simulink model "Trí"  (R2019a)
settings: Solver=FixedStepAuto  StartTime=0.0  StopTime=15  FixedStep=0.01  RelTol=1e-3
model workspace (MATLAB code in the model file):
  | Assem_DataFile.m
undefined symbols (not defined in the file): smiData, X, Y, Z
libraries: sm_lib x272, simulink x8, nesl_utility x8
(part 6 of 6)

== system Trí/Sub_SW/SolidWorks/yoke_haft_arm_8_RIGID ==
  ReferenceFrame : sm_lib/Frames and Transforms/Reference Frame
  Solid : sm_lib/Body Elements/Solid  InertiaType=Custom  Mass=smiData.Solid(6).mass  MassUnits=kg  CenterOfMass=smiData.Solid(6).CoM  CenterOfMassUnits=mm  MomentsOfInertia=smiData.Solid(6).MoI  MomentsOfInertiaUnits=kg*mm^2  ProductsOfInertia=smiData.Solid(6).PoI  ProductsOfInertiaUnits=kg*mm^2  BasedOnType=Density  Density=1000  DensityUnits=kg/m^3  DoExposeReferenceFrame=on  SerializedFrames=<Frames/>  GraphicType=FromGeometry  MarkerShape=Sphere  MarkerSize=10  GraphicVisPropType=SimpleVisualProperties  GraphicDiffuseColor=smiData.Solid(6).color  GraphicSpecularColor=[0.5 0.5 0.5 1.0]  GraphicAmbientColor=[0.15 0.15 0.15 1.0]  GraphicEmissiveColor=[0.0 0.0 0.0 1.0]  GraphicShininess=75  GraphicOpacity=smiData.Solid(6).opacity  GeometryShape=FromFile  RectangleSize=[1 1]  RectangleSizeUnits=m  BrickDimensions=[1 1 1]  BrickDimensionUnits=m  CylinderRadius=1  CylinderRadiusUnits=m  CylinderLength=1  CylinderLengthUnits=m  SphereRadius=1  SphereRadiusUnits=m  EllipsoidRadii=[1 1 1]  EllipsoidRadiiUnits=m  ExtrusionCrossSection=[1 1; -1 1; -1 -1; 1 -1]  ExtrusionCrossSectionUnits=m  ExtrusionLength=1  ExtrusionLengthUnits=m  PolygonNumSides=3  PolygonOuterRadius=1  PolygonOuterRadiusUnits=m  ExtGeomFileType=STEP  ExtGeomFileName=yoke haft arm_Default_sldprt.STEP  ExtGeomFileUnits=m  RevolutionCrossSection=[1 1; 1 -1; 2 -1; 2 1]  RevolutionCrossSectionUnits=m  RevolutionExtent=Full  RevolutionAngle=180  RevolutionAngleUnits=deg
  Transform : sm_lib/Frames and Transforms/Rigid Transform  TranslationMethod=Cartesian  TranslationStandardOffset=0  TranslationLengthUnit=mm  TranslationStandardAxis=+Z  TranslationCartesianOffset=smiData.RigidTransform(66).translation  TranslationROffset=0  TranslationROffsetUnits=m  TranslationZOffset=0  TranslationZOffsetUnits=m  TranslationThetaOffset=0  TranslationThetaOffsetUnits=deg  RotationMethod=ArbitraryAxis  RotationAngleUnits=rad  RotationStandardAxis=+Z  RotationAngle=smiData.RigidTransform(66).angle  RotationArbitraryAxis=smiData.RigidTransform(66).axis  FollAlignAxisA=+X  BaseAlignAxisA=+Y  FollAlignAxisB=+Y  BaseAlignAxisB=+Z  RotationSequenceAxes=FollowerAxes  RotationSequence=XYX  RotationSequenceAngles=[0 0 0]  RotationSequenceAnglesUnits=deg  RotationMatrix=[1 0 0; 0 1 0; 0 0 1]
  Transform1 : sm_lib/Frames and Transforms/Rigid Transform  TranslationMethod=Cartesian  TranslationStandardOffset=0  TranslationLengthUnit=mm  TranslationStandardAxis=+Z  TranslationCartesianOffset=smiData.RigidTransform(121).translation  TranslationROffset=0  TranslationROffsetUnits=m  TranslationZOffset=0  TranslationZOffsetUnits=m  TranslationThetaOffset=0  TranslationThetaOffsetUnits=deg  RotationMethod=ArbitraryAxis  RotationAngleUnits=rad  RotationStandardAxis=+Z  RotationAngle=smiData.RigidTransform(121).angle  RotationArbitraryAxis=smiData.RigidTransform(121).axis  FollAlignAxisA=+X  BaseAlignAxisA=+Y  FollAlignAxisB=+Y  BaseAlignAxisB=+Z  RotationSequenceAxes=FollowerAxes  RotationSequence=XYX  RotationSequenceAngles=[0 0 0]  RotationSequenceAnglesUnits=deg  RotationMatrix=[1 0 0; 0 1 0; 0 0 1]
  F1 : PMIOPort  Side=Left
  F : PMIOPort  Port=2  Side=Left
  connections:
  Solid/RConn1 -- ReferenceFrame/RConn1 -- Transform/LConn1 -- Transform1/LConn1
  Transform/RConn1 -- F/RConn1
  Transform1/RConn1 -- F1/RConn1

== system Trí/Sub_SW/SolidWorks/yoke_haft_arm_9_RIGID ==
  ReferenceFrame : sm_lib/Frames and Transforms/Reference Frame
  Solid : sm_lib/Body Elements/Solid  InertiaType=Custom  Mass=smiData.Solid(6).mass  MassUnits=kg  CenterOfMass=smiData.Solid(6).CoM  CenterOfMassUnits=mm  MomentsOfInertia=smiData.Solid(6).MoI  MomentsOfInertiaUnits=kg*mm^2  ProductsOfInertia=smiData.Solid(6).PoI  ProductsOfInertiaUnits=kg*mm^2  BasedOnType=Density  Density=1000  DensityUnits=kg/m^3  DoExposeReferenceFrame=on  SerializedFrames=<Frames/>  GraphicType=FromGeometry  MarkerShape=Sphere  MarkerSize=10  GraphicVisPropType=SimpleVisualProperties  GraphicDiffuseColor=smiData.Solid(6).color  GraphicSpecularColor=[0.5 0.5 0.5 1.0]  GraphicAmbientColor=[0.15 0.15 0.15 1.0]  GraphicEmissiveColor=[0.0 0.0 0.0 1.0]  GraphicShininess=75  GraphicOpacity=smiData.Solid(6).opacity  GeometryShape=FromFile  RectangleSize=[1 1]  RectangleSizeUnits=m  BrickDimensions=[1 1 1]  BrickDimensionUnits=m  CylinderRadius=1  CylinderRadiusUnits=m  CylinderLength=1  CylinderLengthUnits=m  SphereRadius=1  SphereRadiusUnits=m  EllipsoidRadii=[1 1 1]  EllipsoidRadiiUnits=m  ExtrusionCrossSection=[1 1; -1 1; -1 -1; 1 -1]  ExtrusionCrossSectionUnits=m  ExtrusionLength=1  ExtrusionLengthUnits=m  PolygonNumSides=3  PolygonOuterRadius=1  PolygonOuterRadiusUnits=m  ExtGeomFileType=STEP  ExtGeomFileName=yoke haft arm_Default_sldprt.STEP  ExtGeomFileUnits=m  RevolutionCrossSection=[1 1; 1 -1; 2 -1; 2 1]  RevolutionCrossSectionUnits=m  RevolutionExtent=Full  RevolutionAngle=180  RevolutionAngleUnits=deg
  Transform : sm_lib/Frames and Transforms/Rigid Transform  TranslationMethod=Cartesian  TranslationStandardOffset=0  TranslationLengthUnit=mm  TranslationStandardAxis=+Z  TranslationCartesianOffset=smiData.RigidTransform(55).translation  TranslationROffset=0  TranslationROffsetUnits=m  TranslationZOffset=0  TranslationZOffsetUnits=m  TranslationThetaOffset=0  TranslationThetaOffsetUnits=deg  RotationMethod=ArbitraryAxis  RotationAngleUnits=rad  RotationStandardAxis=+Z  RotationAngle=smiData.RigidTransform(55).angle  RotationArbitraryAxis=smiData.RigidTransform(55).axis  FollAlignAxisA=+X  BaseAlignAxisA=+Y  FollAlignAxisB=+Y  BaseAlignAxisB=+Z  RotationSequenceAxes=FollowerAxes  RotationSequence=XYX  RotationSequenceAngles=[0 0 0]  RotationSequenceAnglesUnits=deg  RotationMatrix=[1 0 0; 0 1 0; 0 0 1]
  Transform1 : sm_lib/Frames and Transforms/Rigid Transform  TranslationMethod=Cartesian  TranslationStandardOffset=0  TranslationLengthUnit=mm  TranslationStandardAxis=+Z  TranslationCartesianOffset=smiData.RigidTransform(70).translation  TranslationROffset=0  TranslationROffsetUnits=m  TranslationZOffset=0  TranslationZOffsetUnits=m  TranslationThetaOffset=0  TranslationThetaOffsetUnits=deg  RotationMethod=ArbitraryAxis  RotationAngleUnits=rad  RotationStandardAxis=+Z  RotationAngle=smiData.RigidTransform(70).angle  RotationArbitraryAxis=smiData.RigidTransform(70).axis  FollAlignAxisA=+X  BaseAlignAxisA=+Y  FollAlignAxisB=+Y  BaseAlignAxisB=+Z  RotationSequenceAxes=FollowerAxes  RotationSequence=XYX  RotationSequenceAngles=[0 0 0]  RotationSequenceAnglesUnits=deg  RotationMatrix=[1 0 0; 0 1 0; 0 0 1]
  Transform2 : sm_lib/Frames and Transforms/Rigid Transform  TranslationMethod=Cartesian  TranslationStandardOffset=0  TranslationLengthUnit=mm  TranslationStandardAxis=+Z  TranslationCartesianOffset=smiData.RigidTransform(119).translation  TranslationROffset=0  TranslationROffsetUnits=m  TranslationZOffset=0  TranslationZOffsetUnits=m  TranslationThetaOffset=0  TranslationThetaOffsetUnits=deg  RotationMethod=ArbitraryAxis  RotationAngleUnits=rad  RotationStandardAxis=+Z  RotationAngle=smiData.RigidTransform(119).angle  RotationArbitraryAxis=smiData.RigidTransform(119).axis  FollAlignAxisA=+X  BaseAlignAxisA=+Y  FollAlignAxisB=+Y  BaseAlignAxisB=+Z  RotationSequenceAxes=FollowerAxes  RotationSequence=XYX  RotationSequenceAngles=[0 0 0]  RotationSequenceAnglesUnits=deg  RotationMatrix=[1 0 0; 0 1 0; 0 0 1]
  F2 : PMIOPort  Side=Left
  F1 : PMIOPort  Port=2  Side=Left
  F : PMIOPort  Port=3  Side=Left
  connections:
  Solid/RConn1 -- ReferenceFrame/RConn1 -- Transform/LConn1 -- Transform1/LConn1 -- Transform2/LConn1
  Transform/RConn1 -- F/RConn1
  Transform1/RConn1 -- F1/RConn1
  Transform2/RConn1 -- F2/RConn1

== system Trí/Sub_SW/SolidWorks/yoke_haft_arm_fake_1_RIGID ==
  ReferenceFrame : sm_lib/Frames and Transforms/Reference Frame
  Solid : sm_lib/Body Elements/Solid  InertiaType=Custom  Mass=smiData.Solid(7).mass  MassUnits=kg  CenterOfMass=smiData.Solid(7).CoM  CenterOfMassUnits=mm  MomentsOfInertia=smiData.Solid(7).MoI  MomentsOfInertiaUnits=kg*mm^2  ProductsOfInertia=smiData.Solid(7).PoI  ProductsOfInertiaUnits=kg*mm^2  BasedOnType=Density  Density=1000  DensityUnits=kg/m^3  DoExposeReferenceFrame=on  SerializedFrames=<Frames/>  GraphicType=FromGeometry  MarkerShape=Sphere  MarkerSize=10  GraphicVisPropType=SimpleVisualProperties  GraphicDiffuseColor=smiData.Solid(7).color  GraphicSpecularColor=[0.5 0.5 0.5 1.0]  GraphicAmbientColor=[0.15 0.15 0.15 1.0]  GraphicEmissiveColor=[0.0 0.0 0.0 1.0]  GraphicShininess=75  GraphicOpacity=smiData.Solid(7).opacity  GeometryShape=FromFile  RectangleSize=[1 1]  RectangleSizeUnits=m  BrickDimensions=[1 1 1]  BrickDimensionUnits=m  CylinderRadius=1  CylinderRadiusUnits=m  CylinderLength=1  CylinderLengthUnits=m  SphereRadius=1  SphereRadiusUnits=m  EllipsoidRadii=[1 1 1]  EllipsoidRadiiUnits=m  ExtrusionCrossSection=[1 1; -1 1; -1 -1; 1 -1]  ExtrusionCrossSectionUnits=m  ExtrusionLength=1  ExtrusionLengthUnits=m  PolygonNumSides=3  PolygonOuterRadius=1  PolygonOuterRadiusUnits=m  ExtGeomFileType=STEP  ExtGeomFileName=yoke haft arm fake_Default_sldprt.STEP  ExtGeomFileUnits=m  RevolutionCrossSection=[1 1; 1 -1; 2 -1; 2 1]  RevolutionCrossSectionUnits=m  RevolutionExtent=Full  RevolutionAngle=180  RevolutionAngleUnits=deg
  Transform : sm_lib/Frames and Transforms/Rigid Transform  TranslationMethod=Cartesian  TranslationStandardOffset=0  TranslationLengthUnit=mm  TranslationStandardAxis=+Z  TranslationCartesianOffset=smiData.RigidTransform(103).translation  TranslationROffset=0  TranslationROffsetUnits=m  TranslationZOffset=0  TranslationZOffsetUnits=m  TranslationThetaOffset=0  TranslationThetaOffsetUnits=deg  RotationMethod=ArbitraryAxis  RotationAngleUnits=rad  RotationStandardAxis=+Z  RotationAngle=smiData.RigidTransform(103).angle  RotationArbitraryAxis=smiData.RigidTransform(103).axis  FollAlignAxisA=+X  BaseAlignAxisA=+Y  FollAlignAxisB=+Y  BaseAlignAxisB=+Z  RotationSequenceAxes=FollowerAxes  RotationSequence=XYX  RotationSequenceAngles=[0 0 0]  RotationSequenceAnglesUnits=deg  RotationMatrix=[1 0 0; 0 1 0; 0 0 1]
  Transform1 : sm_lib/Frames and Transforms/Rigid Transform  TranslationMethod=Cartesian  TranslationStandardOffset=0  TranslationLengthUnit=mm  TranslationStandardAxis=+Z  TranslationCartesianOffset=smiData.RigidTransform(106).translation  TranslationROffset=0  TranslationROffsetUnits=m  TranslationZOffset=0  TranslationZOffsetUnits=m  TranslationThetaOffset=0  TranslationThetaOffsetUnits=deg  RotationMethod=ArbitraryAxis  RotationAngleUnits=rad  RotationStandardAxis=+Z  RotationAngle=smiData.RigidTransform(106).angle  RotationArbitraryAxis=smiData.RigidTransform(106).axis  FollAlignAxisA=+X  BaseAlignAxisA=+Y  FollAlignAxisB=+Y  BaseAlignAxisB=+Z  RotationSequenceAxes=FollowerAxes  RotationSequence=XYX  RotationSequenceAngles=[0 0 0]  RotationSequenceAnglesUnits=deg  RotationMatrix=[1 0 0; 0 1 0; 0 0 1]
  Transform2 : sm_lib/Frames and Transforms/Rigid Transform  TranslationMethod=Cartesian  TranslationStandardOffset=0  TranslationLengthUnit=mm  TranslationStandardAxis=+Z  TranslationCartesianOffset=smiData.RigidTransform(107).translation  TranslationROffset=0  TranslationROffsetUnits=m  TranslationZOffset=0  TranslationZOffsetUnits=m  TranslationThetaOffset=0  TranslationThetaOffsetUnits=deg  RotationMethod=ArbitraryAxis  RotationAngleUnits=rad  RotationStandardAxis=+Z  RotationAngle=smiData.RigidTransform(107).angle  RotationArbitraryAxis=smiData.RigidTransform(107).axis  FollAlignAxisA=+X  BaseAlignAxisA=+Y  FollAlignAxisB=+Y  BaseAlignAxisB=+Z  RotationSequenceAxes=FollowerAxes  RotationSequence=XYX  RotationSequenceAngles=[0 0 0]  RotationSequenceAnglesUnits=deg  RotationMatrix=[1 0 0; 0 1 0; 0 0 1]
  F2 : PMIOPort  Side=Left
  F : PMIOPort  Port=2  Side=Left
  F1 : PMIOPort  Port=3  Side=Left
  connections:
  Solid/RConn1 -- ReferenceFrame/RConn1 -- Transform/LConn1 -- Transform1/LConn1 -- Transform2/LConn1
  Transform/RConn1 -- F/RConn1
  Transform1/RConn1 -- F1/RConn1
  Transform2/RConn1 -- F2/RConn1

== system Trí/Sub_SW/SolidWorks/arm_robot_1_RIGID/Arm_Robot_6_1_RIGID ==
  ReferenceFrame : sm_lib/Frames and Transforms/Reference Frame
  Solid : sm_lib/Body Elements/Solid  InertiaType=Custom  Mass=smiData.Solid(19).mass  MassUnits=kg  CenterOfMass=smiData.Solid(19).CoM  CenterOfMassUnits=mm  MomentsOfInertia=smiData.Solid(19).MoI  MomentsOfInertiaUnits=kg*mm^2  ProductsOfInertia=smiData.Solid(19).PoI  ProductsOfInertiaUnits=kg*mm^2  BasedOnType=Density  Density=1000  DensityUnits=kg/m^3  DoExposeReferenceFrame=on  SerializedFrames=<Frames/>  GraphicType=FromGeometry  MarkerShape=Sphere  MarkerSize=10  GraphicVisPropType=SimpleVisualProperties  GraphicDiffuseColor=smiData.Solid(19).color  GraphicSpecularColor=[0.5 0.5 0.5 1.0]  GraphicAmbientColor=[0.15 0.15 0.15 1.0]  GraphicEmissiveColor=[0.0 0.0 0.0 1.0]  GraphicShininess=75  GraphicOpacity=smiData.Solid(19).opacity  GeometryShape=FromFile  RectangleSize=[1 1]  RectangleSizeUnits=m  BrickDimensions=[1 1 1]  BrickDimensionUnits=m  CylinderRadius=1  CylinderRadiusUnits=m  CylinderLength=1  CylinderLengthUnits=m  SphereRadius=1  SphereRadiusUnits=m  EllipsoidRadii=[1 1 1]  EllipsoidRadiiUnits=m  ExtrusionCrossSection=[1 1; -1 1; -1 -1; 1 -1]  ExtrusionCrossSectionUnits=m  ExtrusionLength=1  ExtrusionLengthUnits=m  PolygonNumSides=3  PolygonOuterRadius=1  PolygonOuterRadiusUnits=m  ExtGeomFileType=STEP  ExtGeomFileName=Arm Robot 6_Default_sldprt.STEP  ExtGeomFileUnits=m  RevolutionCrossSection=[1 1; 1 -1; 2 -1; 2 1]  RevolutionCrossSectionUnits=m  RevolutionExtent=Full  RevolutionAngle=180  RevolutionAngleUnits=deg
  F : PMIOPort  Side=Left
  connections:
  Solid/RConn1 -- ReferenceFrame/RConn1 -- F/RConn1

== system Trí/Sub_SW/SolidWorks/arm_robot_1_RIGID/Arm_Robot_7_1_RIGID ==
  ReferenceFrame : sm_lib/Frames and Transforms/Reference Frame
  Solid : sm_lib/Body Elements/Solid  InertiaType=Custom  Mass=smiData.Solid(20).mass  MassUnits=kg  CenterOfMass=smiData.Solid(20).CoM  CenterOfMassUnits=mm  MomentsOfInertia=smiData.Solid(20).MoI  MomentsOfInertiaUnits=kg*mm^2  ProductsOfInertia=smiData.Solid(20).PoI  ProductsOfInertiaUnits=kg*mm^2  BasedOnType=Density  Density=1000  DensityUnits=kg/m^3  DoExposeReferenceFrame=on  SerializedFrames=<Frames/>  GraphicType=FromGeometry  MarkerShape=Sphere  MarkerSize=10  GraphicVisPropType=SimpleVisualProperties  GraphicDiffuseColor=smiData.Solid(20).color  GraphicSpecularColor=[0.5 0.5 0.5 1.0]  GraphicAmbientColor=[0.15 0.15 0.15 1.0]  GraphicEmissiveColor=[0.0 0.0 0.0 1.0]  GraphicShininess=75  GraphicOpacity=smiData.Solid(20).opacity  GeometryShape=FromFile  RectangleSize=[1 1]  RectangleSizeUnits=m  BrickDimensions=[1 1 1]  BrickDimensionUnits=m  CylinderRadius=1  CylinderRadiusUnits=m  CylinderLength=1  CylinderLengthUnits=m  SphereRadius=1  SphereRadiusUnits=m  EllipsoidRadii=[1 1 1]  EllipsoidRadiiUnits=m  ExtrusionCrossSection=[1 1; -1 1; -1 -1; 1 -1]  ExtrusionCrossSectionUnits=m  ExtrusionLength=1  ExtrusionLengthUnits=m  PolygonNumSides=3  PolygonOuterRadius=1  PolygonOuterRadiusUnits=m  ExtGeomFileType=STEP  ExtGeomFileName=Arm Robot 7_Default_sldprt.STEP  ExtGeomFileUnits=m  RevolutionCrossSection=[1 1; 1 -1; 2 -1; 2 1]  RevolutionCrossSectionUnits=m  RevolutionExtent=Full  RevolutionAngle=180  RevolutionAngleUnits=deg
  F : PMIOPort  Side=Left
  connections:
  Solid/RConn1 -- ReferenceFrame/RConn1 -- F/RConn1

== system Trí/Sub_SW/SolidWorks/arm_robot_1_RIGID/Arm_Robot_8_1_RIGID ==
  ReferenceFrame : sm_lib/Frames and Transforms/Reference Frame
  Solid : sm_lib/Body Elements/Solid  InertiaType=Custom  Mass=smiData.Solid(18).mass  MassUnits=kg  CenterOfMass=smiData.Solid(18).CoM  CenterOfMassUnits=mm  MomentsOfInertia=smiData.Solid(18).MoI  MomentsOfInertiaUnits=kg*mm^2  ProductsOfInertia=smiData.Solid(18).PoI  ProductsOfInertiaUnits=kg*mm^2  BasedOnType=Density  Density=1000  DensityUnits=kg/m^3  DoExposeReferenceFrame=on  SerializedFrames=<Frames/>  GraphicType=FromGeometry  MarkerShape=Sphere  MarkerSize=10  GraphicVisPropType=SimpleVisualProperties  GraphicDiffuseColor=smiData.Solid(18).color  GraphicSpecularColor=[0.5 0.5 0.5 1.0]  GraphicAmbientColor=[0.15 0.15 0.15 1.0]  GraphicEmissiveColor=[0.0 0.0 0.0 1.0]  GraphicShininess=75  GraphicOpacity=smiData.Solid(18).opacity  GeometryShape=FromFile  RectangleSize=[1 1]  RectangleSizeUnits=m  BrickDimensions=[1 1 1]  BrickDimensionUnits=m  CylinderRadius=1  CylinderRadiusUnits=m  CylinderLength=1  CylinderLengthUnits=m  SphereRadius=1  SphereRadiusUnits=m  EllipsoidRadii=[1 1 1]  EllipsoidRadiiUnits=m  ExtrusionCrossSection=[1 1; -1 1; -1 -1; 1 -1]  ExtrusionCrossSectionUnits=m  ExtrusionLength=1  ExtrusionLengthUnits=m  PolygonNumSides=3  PolygonOuterRadius=1  PolygonOuterRadiusUnits=m  ExtGeomFileType=STEP  ExtGeomFileName=Arm Robot 8_Default_sldprt.STEP  ExtGeomFileUnits=m  RevolutionCrossSection=[1 1; 1 -1; 2 -1; 2 1]  RevolutionCrossSectionUnits=m  RevolutionExtent=Full  RevolutionAngle=180  RevolutionAngleUnits=deg
  F : PMIOPort  Side=Left
  connections:
  Solid/RConn1 -- ReferenceFrame/RConn1 -- F/RConn1

== system Trí/Sub_SW/SolidWorks/arm_robot_1_RIGID/x1_2_RIGID ==
  ReferenceFrame : sm_lib/Frames and Transforms/Reference Frame
  Solid : sm_lib/Body Elements/Solid  InertiaType=Custom  Mass=smiData.Solid(21).mass  MassUnits=kg  CenterOfMass=smiData.Solid(21).CoM  CenterOfMassUnits=mm  MomentsOfInertia=smiData.Solid(21).MoI  MomentsOfInertiaUnits=kg*mm^2  ProductsOfInertia=smiData.Solid(21).PoI  ProductsOfInertiaUnits=kg*mm^2  BasedOnType=Density  Density=1000  DensityUnits=kg/m^3  DoExposeReferenceFrame=on  SerializedFrames=<Frames/>  GraphicType=FromGeometry  MarkerShape=Sphere  MarkerSize=10  GraphicVisPropType=SimpleVisualProperties  GraphicDiffuseColor=smiData.Solid(21).color  GraphicSpecularColor=[0.5 0.5 0.5 1.0]  GraphicAmbientColor=[0.15 0.15 0.15 1.0]  GraphicEmissiveColor=[0.0 0.0 0.0 1.0]  GraphicShininess=75  GraphicOpacity=smiData.Solid(21).opacity  GeometryShape=FromFile  RectangleSize=[1 1]  RectangleSizeUnits=m  BrickDimensions=[1 1 1]  BrickDimensionUnits=m  CylinderRadius=1  CylinderRadiusUnits=m  CylinderLength=1  CylinderLengthUnits=m  SphereRadius=1  SphereRadiusUnits=m  EllipsoidRadii=[1 1 1]  EllipsoidRadiiUnits=m  ExtrusionCrossSection=[1 1; -1 1; -1 -1; 1 -1]  ExtrusionCrossSectionUnits=m  ExtrusionLength=1  ExtrusionLengthUnits=m  PolygonNumSides=3  PolygonOuterRadius=1  PolygonOuterRadiusUnits=m  ExtGeomFileType=STEP  ExtGeomFileName=1_Default_sldprt.STEP  ExtGeomFileUnits=m  RevolutionCrossSection=[1 1; 1 -1; 2 -1; 2 1]  RevolutionCrossSectionUnits=m  RevolutionExtent=Full  RevolutionAngle=180  RevolutionAngleUnits=deg
  F : PMIOPort  Side=Left
  connections:
  Solid/RConn1 -- ReferenceFrame/RConn1 -- F/RConn1

== matlab function Trí/Trajectory /Direction path ==
  data: Px output; Py output; Pz output; Alpha output; Beta output; Gama_start input; Gama output; Beta_start input; Alpha_start input; Gama_end input; Beta_end input; Alpha_end input; t input; tf input
function [Px,Py,Pz,Alpha,Beta,Gama]= Direction(Gama_start,Beta_start,Alpha_start,Gama_end,Beta_end,Alpha_end,t,tf)

if mod(t,2*tf)<=tf
   tp = t-floor(t/(2*tf))*2*tf;
   Beta     = Beta_start  + (3/tf^2)*(Beta_end-Beta_start)*tp.^2   - (2/tf^3)*(Beta_end-Beta_start)*tp.^3;
   Gama     = Gama_start  + (3/tf^2)*(Gama_end-Gama_start)*tp.^2   - (2/tf^3)*(Gama_end-Gama_start)*tp.^3;
   Alpha    = Alpha_start + (3/tf^2)*(Alpha_end-Alpha_start)*tp.^2 - (2/tf^3)*(Alpha_end-Alpha_start)*tp.^3;
else
    temp = Beta_start;
    Beta_start = Beta_end;
    Beta_end = temp;
    
    temp = Gama_start;
    Gama_start = Gama_end;
    Gama_end = temp;
    
    temp = Alpha_start;
    Alpha_start = Alpha_end;
    Alpha_end = temp;
    
    tt = t-floor(t/(2*tf))*2*tf-tf;
    Beta  = Beta_start+(3/tf^2)*(Beta_end-Beta_start)*(tt).^2     - (2/tf^3)*(Beta_end-Beta_start)*(tt).^3;
    Gama  = Gama_start+ (3/tf^2)*(Gama_end-Gama_start)*(tt).^2    - (2/tf^3)*(Gama_end-Gama_start)*(tt).^3;
    Alpha = Alpha_start+ (3/tf^2)*(Alpha_end-Alpha_start)*(tt).^2 - (2/tf^3)*(Alpha_end-Alpha_start)*(tt).^3;
end
Px=1178;
Py=0;
Pz=0;
end

== matlab function Trí/CCD Algorithm  ==
  data: Px input; t1 output; Py input; Pz input; alpha input; beta input; gama input; t2 output; t3 output; t4 output; t5 output; t6 output
function [t1,t2,t3,t4,t5,t6]= CCD(Px,Py,Pz,alpha,beta,gama)

%%
L1 = 290.14;
L2 = 360;
L3 = 360;
L4 = 232.87;
%%
theta1 = 60;
theta2 = 60;
theta3 = 60;
theta4 = 60;
theta5 = -60;
theta6 = 60;

%%
% gama = 0; %% R_x
% beta = 0; %% R_y
% alpha = 0; %% R_z
up = [45,45,45,45,45,45];
low = [-45,-30,-45,-30,-45,-45];
%%
ca = cosd(alpha);
sa = sind(alpha);
cb = cosd(beta);
sb = sind(beta);
cg = cosd(gama);
sg = sind(gama);
%% Rotation matrix 1
r11 = ca*cb;
r12 = ca*sb*sg-sa*cg;
r13 = ca*sb*cg+sa*sg;
r21 = sa*cb;
r22 = sa*sb*sg+ca*cg;
r23 = sa*sb*cg-ca*sg;
r31 = -sb;
r32 = cb*sg;
r33 = cb*cg;
% %% Rotation matric 2
% r11 = ca*cb*cg - sa*sg;
% r21 = sa*cb*cg + ca*sg;
% r31 = -sb*cg;
%%
Pf = [Px Py Pz];
Pf_05= [Pf(1)-L4*r11 Pf(2)-L4*r21 Pf(3)-L4*r31];


%% vi tri T05
Pe_x = L1 + L2*cosd(theta1)*cosd(theta2) - L3*cosd(theta4)*(sind(theta1)*sind(theta3) - cosd(theta1)*cosd(theta2)*cosd(theta3)) - L3*cosd(theta1)*sind(theta2)*sind(theta4);
Pe_y = L2*cosd(theta2)*sind(theta1) + L3*cosd(theta4)*(cosd(theta1)*sind(theta3) + cosd(theta2)*cosd(theta3)*sind(theta1)) - L3*sind(theta1)*sind(theta2)*sind(theta4);
Pe_z = L2*sind(theta2) + L3*cosd(theta2)*sind(theta4) + L3*cosd(theta3)*cosd(theta4)*sind(theta2);
Pe = [Pe_x Pe_y Pe_z];
%%
A1 = distance_246(Pe,Pf_05);
A2 = distance_135(Pe,Pf_05);

while ((A1>0.01)||(A2>0.01))
    %% Pc2 
    Pc2_x = L1 + L2*cosd(theta1)*cosd(theta2);    % T03
    Pc2_y = L2*cosd(theta2)*sind(theta1);
    Pc2_z = L2*sind(theta2);
    Pc2 = [Pc2_x Pc2_y Pc2_z];
    B = Calculate_246(Pe,Pc2,Pf_05);
    theta = B(1);
    Z = B(2);
    theta4 = Z*theta+theta4;
    theta4 = scale_value(theta4,up(4),low(4));
    Pe = Rotation_theta4(theta1,theta2,theta3,theta4,L1,L2,L3,L4);
    %% Pc1
    Pc1 = [L1 0 0];
    B = Calculate_246(Pe,Pc1,Pf_05);
    theta = B(1);
    Z = B(2);
    theta2 = Z*theta+theta2;
    theta2 = scale_value(theta2,up(2),low(2));
    Pe = Rotation_theta2(theta1,theta2,theta3,theta4,L1,L2,L3,L4);
    %% tinh khoang cach
    A1 = distance_246(Pe,Pf_05);
    Pe = [Pe(1) Pe(2) Pe(3)];
    %% Pc2
    Pc2_x = L1 + L2*cosd(theta1)*cosd(theta2);    % T03
    Pc2_y = L2*cosd(theta2)*sind(theta1);
    Pc2_z = L2*sind(theta2);
    Pc2 = [Pc2_x Pc2_y Pc2_z];
    B = Calculate_135(Pe,Pc2,Pf_05);
    theta = B(1);
    Z = B(2);
    theta3 = Z*theta+theta3;
    theta3 = scale_value(theta3,up(3),low(3));
    Pe = Rotation_theta3(theta1,theta2,theta3,theta4,L1,L2,L3,L4);
    %% Pc1
    Pc1 = [L1 0 0];
    B = Calculate_135(Pe,Pc1,Pf_05);
    theta = B(1);
    Z = B(2);
    theta1 = Z*theta+theta1;
    theta1 = scale_value(theta1,up(1),low(1));
    Pe = Rotation_theta1(theta1,theta2,theta3,theta4,L1,L2,L3,L4);
    %% tinh khoang cach
    A2 = distance_135(Pe,Pf_05);
    Pe = [Pe(1) Pe(2) Pe(3)];   
end
%% vi tri T07
Pe_x = L1 + L2*cosd(theta1)*cosd(theta2) + L4*sind(theta6)*(sind(theta4)*(sind(theta1)*sind(theta3) - cosd(theta1)*cosd(theta2)*cosd(theta3)) - cosd(theta1)*cosd(theta4)*sind(theta2)) - L4*cosd(theta6)*(cosd(theta5)*(cosd(theta4)*(sind(theta1)*sind(theta3) - cosd(theta1)*cosd(theta2)*cosd(theta3)) + cosd(theta1)*sind(theta2)*sind(theta4)) + sind(theta5)*(cosd(theta3)*sind(theta1) + cosd(theta1)*cosd(theta2)*sind(theta3))) - L3*cosd(theta4)*(sind(theta1)*sind(theta3) - cosd(theta1)*cosd(theta2)*cosd(theta3)) - L3*cosd(theta1)*sind(theta2)*sind(theta4); 
Pe_y = L2*cosd(theta2)*sind(theta1) - L4*sind(theta6)*(sind(theta4)*(cosd(theta1)*sind(theta3) + cosd(theta2)*cosd(theta3)*sind(theta1)) + cosd(theta4)*sind(theta1)*sind(theta2)) + L3*cosd(theta4)*(cosd(theta1)*sind(theta3) + cosd(theta2)*cosd(theta3)*sind(theta1)) + L4*cosd(theta6)*(cosd(theta5)*(cosd(theta4)*(cosd(theta1)*sind(theta3) + cosd(theta2)*cosd(theta3)*sind(theta1)) - sind(theta1)*sind(theta2)*sind(theta4)) + sind(theta5)*(cosd(theta1)*cosd(theta3) - cosd(theta2)*sind(theta1)*sind(theta3))) - L3*sind(theta1)*sind(theta2)*sind(theta4);
Pe_z = L2*sind(theta2) + L4*sind(theta6)*(cosd(theta2)*cosd(theta4) - cosd(theta3)*sind(theta2)*sind(theta4)) + L3*cosd(theta2)*sind(theta4) + L4*cosd(theta6)*(cosd(theta5)*(cosd(theta2)*sind(theta4) + cosd(theta3)*cosd(theta4)*sind(theta2)) - sind(theta2)*sind(theta3)*sind(theta5)) + L3*cosd(theta3)*cosd(theta4)*sind(theta2);
Pe = [Pe_x Pe_y Pe_z]; 
A1 = distance_246(Pe,Pf);
A2 = distance_135(Pe,Pf);
while ((A1>0.01)||(A2>0.01))
    %% Pc3 frame 246
    Pc3_x = L1 + L2*cosd(theta1)*cosd(theta2) - L3*cosd(theta4)*(sind(theta1)*sind(theta3) - cosd(theta1)*cosd(theta2)*cosd(theta3)) - L3*cosd(theta1)*sind(theta2)*sind(theta4);
    Pc3_y = L2*cosd(theta2)*sind(theta1) + L3*cosd(theta4)*(cosd(theta1)*sind(theta3) + cosd(theta2)*cosd(theta3)*sind(theta1)) - L3*sind(theta1)*sind(theta2)*sind(theta4);
    Pc3_z = L2*sind(theta2) + L3*cosd(theta2)*sind(theta4) + L3*cosd(theta3)*cosd(theta4)*sind(theta2);
    Pc3 = [Pc3_x Pc3_y Pc3_z];
    B = Calculate_246(Pe,Pc3,Pf);
    theta = B(1);
    Z = B(2);
    theta6 = Z*theta+theta6;
    theta6 = scale_value(theta6,up(6),low(6));
    %% tinh khoang cach
    Pe = Rotation_theta6(theta1,theta2,theta3,theta4,theta5,theta6,L1,L2,L3,L4);
    A1 = distance_246(Pe,Pf);
     %% Pc3 frame 135
    Pc3_x = L1 + L2*cosd(theta1)*cosd(theta2) - L3*cosd(theta4)*(sind(theta1)*sind(theta3) - cosd(theta1)*cosd(theta2)*cosd(theta3)) - L3*cosd(theta1)*sind(theta2)*sind(theta4);
    Pc3_y = L2*cosd(theta2)*sind(theta1) + L3*cosd(theta4)*(cosd(theta1)*sind(theta3) + cosd(theta2)*cosd(theta3)*sind(theta1)) - L3*sind(theta1)*sind(theta2)*sind(theta4);
    Pc3_z = L2*sind(theta2) + L3*cosd(theta2)*sind(theta4) + L3*cosd(theta3)*cosd(theta4)*sind(theta2);
    Pc3 = [Pc3_x Pc3_y Pc3_z];
    B = Calculate_135(Pe,Pc3,Pf);
    theta = B(1);
    Z = B(2);
    theta5 = Z*theta+theta5;
    theta5 = scale_value(theta5,up(5),low(5));
    %% tinh khoang cach
    Pe = Rotation_theta5(theta1,theta2,theta3,theta4,theta5,theta6,L1,L2,L3,L4);    
    A2 = distance_135(Pe,Pf);
end
t1 = theta1;
t2 = theta2;
t3 = theta3;
t4 = theta4;
t5 = theta5;
t6 = theta6;

== matlab function Trí/Trajectory /Triangle path ==
  data: Px1 input; Py1 input; Px output; Py output; Pz output; Pz1 input; Px2 input; Py2 input; Pz2 input; Px3 input; Py3 input; Pz3 input; t input; tf input; Anpha output; Beta output; Gama output

function [Px,Py,Pz,Anpha,Beta,Gama]= Triangle(Px1,Py1,Pz1,Px2,Py2,Pz2,Px3,Py3,Pz3,t,tf)

if mod(t,3*tf)<=tf
   tp = t-floor(t/(3*tf))*3*tf;
   Pz = Pz1+(3/tf^2)*(Pz2-Pz1)*tp.^2 - (2/tf^3)*(Pz2-Pz1)*tp.^3;
   Px = Px1+ (3/tf^2)*(Px2-Px1)*tp.^2 - (2/tf^3)*(Px2-Px1)*tp.^3;
   Py = Py1+ (3/tf^2)*(Py2-Py1)*tp.^2 - (2/tf^3)*(Py2-Py1)*tp.^3;
   
else if ((mod(t,3*tf)>tf) && (mod(t,3*tf)<=2*tf))
   tp = t-floor(t/(3*tf))*3*tf-tf;
   Pz = Pz2+(3/tf^2)*(Pz3-Pz2)*tp.^2 - (2/tf^3)*(Pz3-Pz2)*tp.^3;
   Px = Px2+ (3/tf^2)*(Px3-Px2)*tp.^2 - (2/tf^3)*(Px3-Px2)*tp.^3;        
   Py = Py2+ (3/tf^2)*(Py3-Py2)*tp.^2 - (2/tf^3)*(Py3-Py2)*tp.^3;     
        
    else
    tt = t-floor(t/(3*tf))*3*tf-2*tf;
    Pz = Pz3+(3/tf^2)*(Pz1-Pz3)*(tt).^2 - (2/tf^3)*(Pz1-Pz3)*(tt).^3;
    Px = Px3+ (3/tf^2)*(Px1-Px3)*(tt).^2 - (2/tf^3)*(Px1-Px3)*(tt).^3;
    Py = Py3+ (3/tf^2)*(Py1-Py3)*(tt).^2 - (2/tf^3)*(Py1-Py3)*(tt).^3;
    end
end

Anpha=0;
Beta=0;
Gama=0;
end

== matlab function Trí/Trajectory /Line path ==
  data: Px0 input; Px output; Py output; Pz output; Pz0 input; Pxf input; Pzf input; t input; tf input; Anpha output; Beta output; Gama output

function [Px,Py,Pz,Anpha,Beta,Gama]= Line(Px0,Pz0,Pxf,Pzf,t,tf)

if mod(t,2*tf)<=tf
    
   tp = t-floor(t/(2*tf))*2*tf;
   
   Pz = Pz0+(3/tf^2)*(Pzf-Pz0)*tp.^2 - (2/tf^3)*(Pzf-Pz0)*tp.^3;
   Px = Px0+(3/tf^2)*(Pxf-Px0)*tp.^2 - (2/tf^3)*(Pxf-Px0)*tp.^3;
else
    temp = Pz0;
    Pz0 = Pzf;
    Pzf = temp;
    
    tt = t-floor(t/(2*tf))*2*tf-tf;
    
    Pz = Pz0+(3/tf^2)*(Pzf-Pz0)*(tt).^2 - (2/tf^3)*(Pzf-Pz0)*(tt).^3;
    Px = Px0+(3/tf^2)*(Pxf-Px0)*(tt).^2 - (2/tf^3)*(Pxf-Px0)*(tt).^3;
end

Py = 0;
Anpha=0;
Beta=0;
Gama=0;
end

== matlab function Trí/Trajectory /Circle path ==
  data: Px output; tf input; t input; O input; Py output; Pz output; BK input; Alpha output; Beta output; Gama output
function [Px,Py,Pz,Alpha,Beta,Gama] =  Circle(tf,t,O,BK)

Px=1160;
m=20;
A=O(1,1);
B=O(2,1);
P=eye(21);
R=BK;
n = 3;
for i=1:(m+1)
    P(i,1)=A+sin(i*2*pi/m)*R;
    P(i,2)=B+cos(i*2*pi/m)*R;
end
if (t<(n*tf*m))
     i=((mod(t,m*tf)-mod(t,tf))/tf)+1;
     V11=((mod(1,m*tf)-mod(1,tf))/tf)*2*pi/m*cos(i*2*pi/m)*R;
     V21=((mod(1,m*tf)-mod(1,tf))/tf)*2*pi/m*cos((i+1)*2*pi/m)*R;
     V12=-((mod(1,m*tf)-mod(1,tf))/tf)*2*pi/m*sin(i*2*pi/m)*R;
     V22=-((mod(1,m*tf)-mod(1,tf))/tf)*2*pi/m*sin((i+1)*2*pi/m)*R;
     
     Py = P(i,1) + V11*(mod(t,tf*m)-(i-1)*tf).^1 + ((3*P(i+1,1))/tf^2 - (3*P(i,1))/tf^2 - (2*V11)/tf - V21/tf)*(mod(t,tf*m)-(i-1)*tf).^2 + ...
        ((2*P(i,1))/tf^3 - (2*P(i+1,1))/tf^3 + V11/tf^2 + V21/tf^2)*(mod(t,tf*m)-(i-1)*tf).^3;
     Pz = P(i,2) + V12*(mod(t,tf*m)-(i-1)*tf).^1 + ((3*P(i+1,2))/tf^2 - (3*P(i,2))/tf^2 - (2*V12)/tf - V22/tf)*(mod(t,tf*m)-(i-1)*tf).^2 + ...
        ((2*P(i,2))/tf^3 - (2*P(i+1,2))/tf^3 + V12/tf^2 + V22/tf^2)*(mod(t,tf*m)-(i-1)*tf).^3;
else
    Py=P(1,1);
    Pz=P(1,2);
end
Alpha=0;
Beta=0;
Gama=0;
end

== matlab function Trí/Observation/Forward kinematic  ==
  data: theta1 input; Px_FK output; Py_FK output; Pz_FK output; theta2 input; theta3 input; theta4 input; theta5 input; theta6 input; Alpha_FK output; Beta_FK output; Gama_FK output
function [Px_FK,Py_FK,Pz_FK,Alpha_FK,Beta_FK,Gama_FK]= FK(theta1,theta2,theta3,theta4,theta5,theta6)
L1 = 290.14;
L2 = 360;
L3 = 360;
L4 = 232.87;
KQ = forward_kinematic(theta1,theta2,theta3,theta4,theta5,theta6,L1,L2,L3,L4);
Px_FK = KQ(1);
Py_FK = KQ(2);
Pz_FK = KQ(3);
Gama_FK  = KQ(4);
Beta_FK  = KQ(5);
Alpha_FK = KQ(6);
end
